simulink model "MatlabFunc"  (R2020a)
settings: Solver=VariableStepAuto  StartTime=0.0  StopTime=100  RelTol=1e-6
undefined symbols (not defined in the file or in its folder): a1, a2, g, k, m
settings Model: Creator=faith  LastModifiedBy=faith

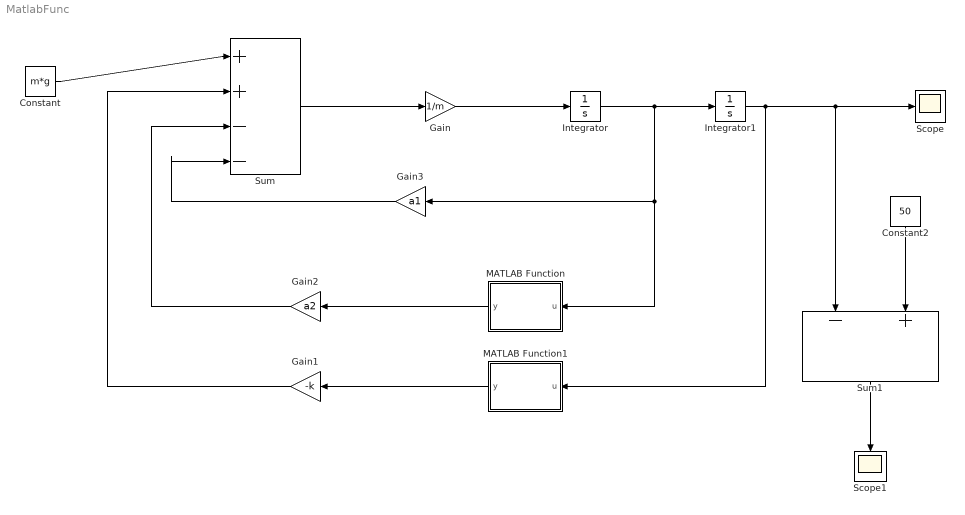
== system MatlabFunc ==
  Constant : Constant  Value=m*g
  Constant2 : Constant  Value=50
  Gain : Gain  Gain=1/m
  Gain1 : Gain  Gain=-k
  Gain2 : Gain  Gain=a2
  Gain3 : Gain  Gain=a1
  Integrator : Integrator
  Integrator1 : Integrator  InitialCondition=-30
  MATLAB Function : MATLAB Function  TreatAsAtomicUnit=on
  MATLAB Function1 : MATLAB Function  TreatAsAtomicUnit=on
  Scope : Scope
  Scope1 : Scope
  Sum : Sum  Inputs=|++--
  Sum1 : Sum  Inputs=-+
  wires:
  Gain3/1 -> Sum/4
  Integrator1/1 -> Scope/1, Sum1/1, MATLAB Function1/1(u)
  Constant/1 -> Sum/1
  Sum/1 -> Gain/1
  Constant2/1 -> Sum1/2
  Sum1/1 -> Scope1/1
  Gain2/1 -> Sum/3
  Gain/1 -> Integrator/1
  Integrator/1 -> MATLAB Function/1(u), Gain3/1, Integrator1/1
  MATLAB Function/1(y) -> Gain2/1
  MATLAB Function1/1(y) -> Gain1/1
  Gain1/1 -> Sum/2

== matlab function MatlabFunc/MATLAB Function ==
  data: u input; y output
function y = fcn(u)
y = abs(u)*u;
end

== matlab function MatlabFunc/MATLAB Function1 ==
  data: u input; y output
function y = fcn(u)
%#codegen
if(u>0)
    y=u;
else
    y=0;
end
end
